simulink model "aufgabe2_sim"  (R2016b)
settings: Solver=VariableStepAuto  StartTime=0.0  StopTime=14  RelTol=1e-3
values from neighbouring files (symbols this model uses):
  A = double([0, 1, -1; -3411/62, -54163/28520, 1/1240;      6822/325, 1/3250, 54117/74750 - (7*1130385^(1/2))/7475])    [aufgabe1.m]    (also in aufgabe2.m; aufgabe4.m; aufgabe5.m; aufgabe6.m)
  bu = double([0; 12500/713; 0])    [aufgabe1.m]    (also in aufgabe2.m; aufgabe4.m; aufgabe5.m; aufgabe6.m)
  ct = [0 0 1]    [aufgabe1.m]    (also in aufgabe2.m; aufgabe4.m; aufgabe5.m; aufgabe6.m = eye(3))
  ct2 = double(subs([0 0 0 1], paralist_1, paralist_2))    [aufgabe2.m]
  g = 0.165707650406087    (= 0.165707650406)    [aufgabe2.m]
  g2 = 1 / ((ct2 + d2*kt2)*inv(eye(4) - phi2 - gamma2*kt2)*gamma2 + d2)    [aufgabe2.m]
  kt = [1.894974536721893,-0.520134683695267,0.478777536929102]    [aufgabe2.m]
  kt2 = -acker(phi2, gamma2, Pd)    [aufgabe2.m]
  Ta = 10e-03    (= 0.01)    [aufgabe1.m]    (also in aufgabe2.m; aufgabe4.m; aufgabe5.m; aufgabe6.m)
  u_GSM_r = 5.6    [aufgabe2.m]    (also in aufgabe4.m; aufgabe6.m; aufgabe7.m)
  x_R = [5.52282806081939;0.506027297604110;30.5949909202308;30.5949909202308]    [aufgabe2.m]
libraries: simulink x1
settings Model: Creator=M  LastModifiedBy=M

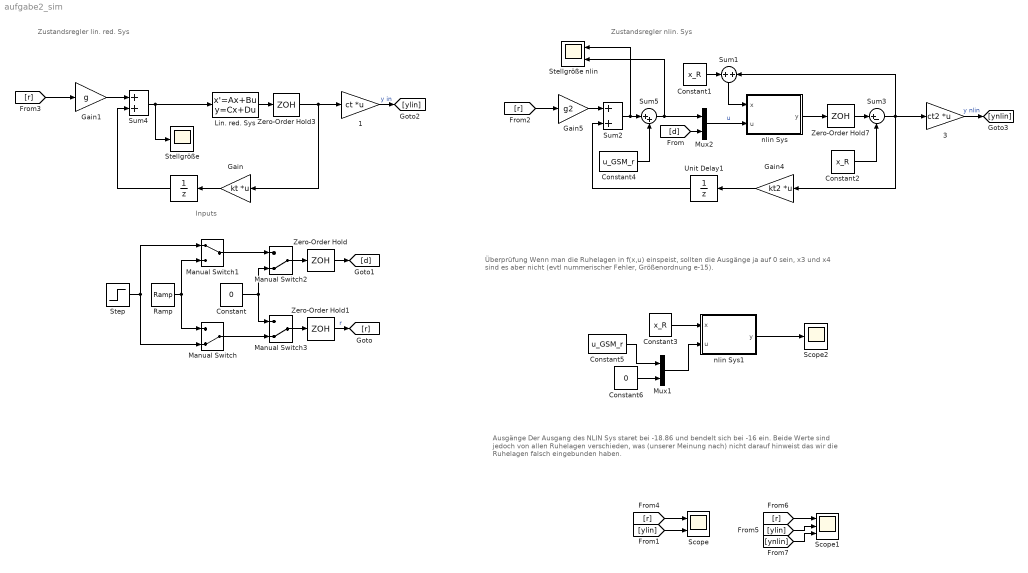
== system aufgabe2_sim ==
  note: Inputs
  note: Zustandsregler lin. red. Sys
  note: Zustandsregler nlin. Sys
  note: Überprüfung
      | Wenn man die Ruhelagen in f(x,u) einspeist, sollten die Ausgänge ja auf 0 sein, x3 und x4 sind es aber nicht (evtl nummerischer Fehler, Größenordnung e-15).
  note: Ausgänge
      | Der Ausgang des NLIN Sys staret bei -18.86 und bendelt sich bei -16 ein. Beide Werte sind jedoch von allen Ruhelagen verschieden, was (unserer Meinung nach) nicht darauf hinweist das wir die Ruhelagen falsch eingebunden haben.
  "  " : UnitDelay  SampleTime=-1
  "   1" : Gain  Gain=ct  Multiplication=Matrix(K*u)
  "   3" : Gain  Gain=ct2  Multiplication=Matrix(K*u)
  Constant : Constant  Value=0
  Constant1 : Constant  Value=x_R
  Constant2 : Constant  Value=x_R
  Constant3 : Constant  Value=x_R
  Constant4 : Constant  Value=u_GSM_r
  Constant5 : Constant  Value=u_GSM_r
  Constant6 : Constant  Value=0
  Gain : Gain  Gain=kt  Multiplication=Matrix(K*u)  SampleTime=Ta
  Gain1 : Gain  Gain=g  SampleTime=Ta
  Gain4 : Gain  Gain=kt2  Multiplication=Matrix(K*u)  SampleTime=Ta
  Gain5 : Gain  Gain=g2  SampleTime=Ta
  Lin. red. Sys : StateSpace  A=A  B=bu  C=eye(3)  D=[0; 0 ; 0]  X0=[0,0,0]
  Manual Switch : ManualSwitch  CurrentSetting=0
  Manual Switch1 : ManualSwitch
  Manual Switch2 : ManualSwitch  CurrentSetting=0
  Manual Switch3 : ManualSwitch  CurrentSetting=0
  Mux1 : Mux  Inputs=2
  Mux2 : Mux  Inputs=2
  Ramp : simulink/Sources/Ramp  slope=1  start=1  X0=0
  Scope : Scope  NumInputPorts=2
  Scope1 : Scope  NumInputPorts=3
  Scope2 : Scope
  Stellgröße : Scope
  Stellgröße nlin : Scope  NumInputPorts=2
  Step : Step  Time=5  SampleTime=0
  Sum1 : Sum
  Sum2 : Sum
  Sum3 : Sum  Inputs=|+-
  Sum4 : Sum
  Sum5 : Sum  Inputs=|++
  Unit Delay1 : UnitDelay  SampleTime=-1
  Zero-Order Hold{,1,3,7} (4 alike) : ZeroOrderHold  SampleTime=Ta
  nlin Sys : MATLAB Function  TreatAsAtomicUnit=on
  nlin Sys1 : MATLAB Function  TreatAsAtomicUnit=on
  wires:
  Manual Switch1/1 -> Manual Switch2/1
  Constant/1 -> Manual Switch3/1, Manual Switch2/2
  Manual Switch2/1 -> Zero-Order Hold/1
  Manual Switch3/1 -> Zero-Order Hold1/1
  Manual Switch/1 -> Manual Switch3/2
  Ramp/1 -> Manual Switch/1, Manual Switch1/2
  Step/1 -> Manual Switch/2, Manual Switch1/1
  Zero-Order Hold1/1 -> [r]  "r"
  Zero-Order Hold/1 -> [d]
  Sum4/1 -> Lin. red. Sys/1, Stellgröße/1
  [r] -> Gain1/1
  Gain1/1 -> Sum4/1
  Gain/1 -> "  "/1
  Lin. red. Sys/1 -> Zero-Order Hold3/1
  Zero-Order Hold3/1 -> Gain/1, "   1"/1
  Gain5/1 -> Sum2/1
  [d] -> Mux2/2
  Gain4/1 -> Unit Delay1/1
  "  "/1 -> Sum4/2
  Sum1/1 -> nlin Sys/1(x)
  Constant1/1 -> Sum1/1
  Zero-Order Hold7/1 -> Sum3/1
  "   1"/1 -> [ylin]  "y in"
  [ylin] -> Scope/2
  [r] -> Scope/1
  [r] -> Scope1/1
  [ylin] -> Scope1/2
  [ynlin] -> Scope1/3
  "   3"/1 -> [ynlin]  "y nlin"
  Mux2/1 -> nlin Sys/2(u)  "u"
  Sum3/1 -> Gain4/1, Sum1/2, "   3"/1
  [r] -> Gain5/1
  nlin Sys/1(y) -> Zero-Order Hold7/1
  Sum2/1 -> Stellgröße nlin/1, Sum5/1
  Sum5/1 -> Mux2/1, Stellgröße nlin/2
  Constant4/1 -> Sum5/2
  Constant2/1 -> Sum3/2
  Unit Delay1/1 -> Sum2/2
  nlin Sys1/1(y) -> Scope2/1
  Constant3/1 -> nlin Sys1/1(x)
  Mux1/1 -> nlin Sys1/2(u)
  Constant5/1 -> Mux1/1
  Constant6/1 -> Mux1/2

== matlab function aufgabe2_sim/nlin Sys1 ==
  data: x input; u input; y output
function y = fcn(x, u)
y = zeros(4, 1);
% Signale auslesen
u_GSM    = u(1);
M_ext    = u(2);
i_GSM    = x(1);
phi_GSMP = x(2);
w_GSM    = x(3);
w_P      = x(4);

f_M_v = [(5000*u_GSM)/7 - (2300*i_GSM)/7 - (500*w_GSM)/7;...
     w_GSM - w_P;...
     (250*i_GSM)/31 - (3411*phi_GSMP)/62 - (181*w_GSM)/1240 + w_P/1240 - 380/31;...
     - w_P^2/325 - (271*w_P)/3250 - (400*M_ext)/13 + (6822*phi_GSMP)/325 + w_GSM/3250 - 26/5];
 
y = double(f_M_v);

== matlab function aufgabe2_sim/nlin Sys ==
  data: x input; u input; y output
function y = fcn(x, u)
y = zeros(4, 1);
% Signale auslesen
u_GSM    = u(1);
M_ext    = u(2);
i_GSM    = x(1);
phi_GSMP = x(2);
w_GSM    = x(3);
w_P      = x(4);

f_M_v = [(5000*u_GSM)/7 - (2300*i_GSM)/7 - (500*w_GSM)/7;...
     w_GSM - w_P;...
     (250*i_GSM)/31 - (3411*phi_GSMP)/62 - (181*w_GSM)/1240 + w_P/1240 - 380/31;...
     - w_P^2/325 - (271*w_P)/3250 - (400*M_ext)/13 + (6822*phi_GSMP)/325 + w_GSM/3250 - 26/5];

y = double(f_M_v);
